simulink model "HW2Simulink"  (R2022a)
settings: Solver=VariableStepAuto  StartTime=0.0  StopTime=1  RelTol=1e-3
model workspace (MAT data in the model file):
  SNR = 15
  SampleTime = 0.001001001001
libraries: commrandsrc3 x2, dspxfrm3 x1, commdigbbndam3 x1
settings Model: PacingRate=1000  Creator=Sander  LastModifiedBy=Sander
settings SolverCC: AlgebraicLoopSolver=TrustRegion
settings DebuggingCC: UnconnectedInputMsg=warning  UnconnectedOutputMsg=warning  UnconnectedLineMsg=warning  SFMachineParentedDataDiag=warning
settings RTWCC: DLArmComputeVersion=19.05

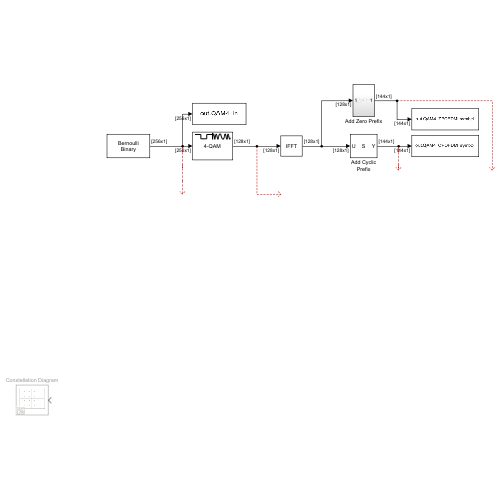
[thumbnail: Simulink's stored preview of the top-level diagram]
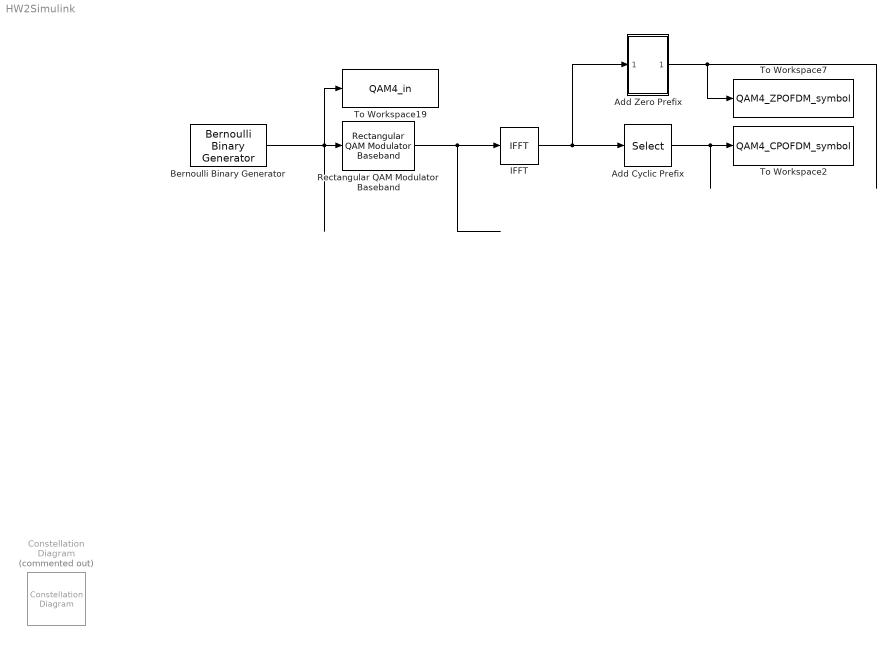
== system HW2Simulink ==
  Add Cyclic Prefix : Selector  InputPortWidth=128  IndexOptions=Index vector (dialog)  Indices=[113:128 1:128]  OutputSizes=1
  Add Zero Prefix : Subsystem
  Bernoulli Binary Generator : commrandsrc3/Bernoulli Binary Generator  ProbabilityOfZero=0.5  SeedSource=Auto  Seed=0  SampleTime=SampleTime  SamplesPerFrame=128*2  OutputDataType=double  SimulateUsing=Interpreted execution
  Constellation Diagram : ConstellationDiagram  Commented=on  WindowPosition=[1.000000,41.000000,1280.000000,657.000000,]  ScopeFrameLocation=window  DefaultConfigurationName=comm.scopes.ConstellationDiagramBlockCfg
  IFFT : dspxfrm3/IFFT  FFTImplementation=Auto  CompMethod=Table lookup  TableOpt=NEW  TableOptActive=Speed  BitRevOrder=off  cs_in=off  Normalize=on  InheritFFTLength=on  FFTLength=64  WrapInput=on  mode=Complex  outSamplingMode=Sample based  roundingMode=Floor  overflowMode=off  firstCoeffDataTypeStr=Inherit: Same word length as input  firstCoeffLastDataTypeStr=Inherit: Same word length as input  outputMin=[]  outputMax=[]
  Rectangular QAM Modulator Baseband : commdigbbndam3/Rectangular QAM Modulator Baseband  M=4  InType=Bit  Enc=Gray  Mapping=[0:15]  PowType=Average Power  MinDist=2  AvgPow=1  PeakPow=1  Ph=0  outDtype=double  outWordLen=16  outUDDataType=sfix(16)  outFracLenMode=Best precision  outFracLen=15  outDataTypeStr=double  outLastDataTypeStr=double
  To Workspace19 : ToWorkspace  VariableName=QAM4_in  SampleTime=SampleTime
      settings: Save2DSignal=2-D array (concatenate along first dimension)
  To Workspace2 : ToWorkspace  VariableName=QAM4_CPOFDM_symbol  SampleTime=SampleTime
      settings: Save2DSignal=2-D array (concatenate along first dimension)
  To Workspace7 : ToWorkspace  VariableName=QAM4_ZPOFDM_symbol  SampleTime=SampleTime
      settings: Save2DSignal=2-D array (concatenate along first dimension)
  wires:
  Bernoulli Binary Generator/1 -> To Workspace19/1, Rectangular QAM Modulator Baseband/1
  Rectangular QAM Modulator Baseband/1 -> IFFT/1
  IFFT/1 -> Add Cyclic Prefix/1, Add Zero Prefix/1(In1)
  Add Cyclic Prefix/1 -> To Workspace2/1
  Add Zero Prefix/1(Out1) -> To Workspace7/1

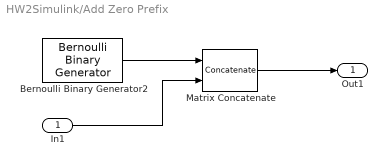
== system HW2Simulink/Add Zero Prefix ==
  In1 : Inport
  Bernoulli Binary Generator2 : commrandsrc3/Bernoulli Binary Generator  ProbabilityOfZero=1  SeedSource=Auto  Seed=0  SampleTime=SampleTime  SamplesPerFrame=16  OutputDataType=double  SimulateUsing=Interpreted execution
  Matrix Concatenate : Concatenate  ConcatenateDimension=2
  Out1 : Outport
  wires:
  Bernoulli Binary Generator2/1 -> Matrix Concatenate/1
  Matrix Concatenate/1 -> Out1/1
  In1/1 -> Matrix Concatenate/2
